simulink model "readFromMat"  (Simulink 8.5)
settings: Solver=ode3  StartTime=0.0  StopTime=100  FixedStep=0.01  RelTol=1e-3
settings Model: Creator=shawn  LastModifiedBy=shawn
settings DataIOCC: SignalLoggingSaveFormat=Dataset
settings OptimizationCC: ExpressionDepthLimit=128
settings DebuggingCC: UnderspecifiedInitializationDetection=Simplified  MergeDetectMultiDrivingBlocksExec=error  FcnCallInpInsideContextMsg=EnableAllAsError  StateNameClashWarn=none
settings GRTTargetCC: CombineOutputUpdateFcns=on  GRTInterface=off

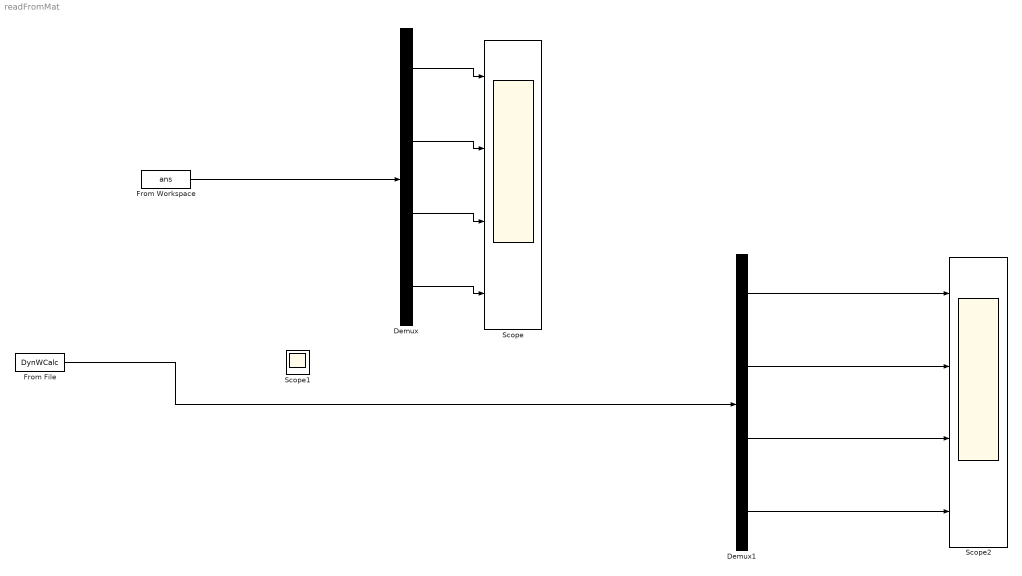
== system readFromMat ==
  Demux : Demux
  Demux1 : Demux
  From Workspace : FromWorkspace  VariableName=ans  SampleTime=0
  From File : FromFile  FileName=DynWCalc  SampleTime=0
  Scope : Scope  NumInputPorts=4
      settings: YMin=-5~-5~-5~-5  YMax=5~5~5~5
  Scope1 : Scope
  Scope2 : Scope  NumInputPorts=4
      settings: YMin=-5~-5~-5~-5  YMax=5~5~5~5  SaveName=ScopeData2
  wires:
  From Workspace/1 -> Demux/1
  Demux/2 -> Scope/2
  Demux/1 -> Scope/1
  Demux/3 -> Scope/3
  Demux/4 -> Scope/4
  From File/1 -> Demux1/1
  Demux1/3 -> Scope2/3
  Demux1/4 -> Scope2/4
  Demux1/2 -> Scope2/2
  Demux1/1 -> Scope2/1
